simulink model "Lab2_TopolnitskiiA_R31342020c_slx"  (R2020b)
settings: Solver=VariableStepAuto  StartTime=0.0  StopTime=10.0  RelTol=1e-3
libraries: roblocks x4, simulink x3
settings Model: Creator=Insight  LastModifiedBy=Insight
settings DebuggingCC: SFMachineParentedDataDiag=error

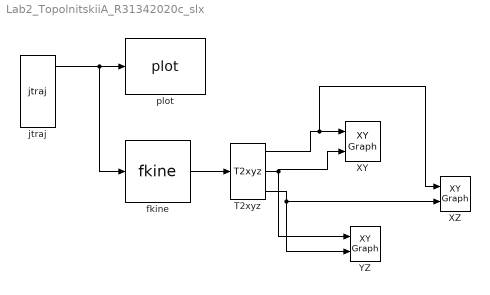
== system Lab2_TopolnitskiiA_R31342020c_slx ==
  T2xyz : roblocks/Toolbox/T2xyz
  XY : simulink/Sinks/XY Graph  xmin=-1  xmax=1  ymin=-1  ymax=1  st=-1
  XZ : simulink/Sinks/XY Graph  xmin=-1.5  xmax=1.5  ymin=-1.5  ymax=1.5  st=-1
  "YZ " : simulink/Sinks/XY Graph  xmin=-1.5  xmax=1.5  ymin=-1.5  ymax=1.5  st=-1
  fkine : roblocks/Arm/fkine  robot=irb140
  jtraj : roblocks/Toolbox/jtraj  q0=[pi/4 pi/4 pi/10 pi/10 pi/15 pi/5]  qf=[-pi/4 -6*pi/7 pi/2 -pi -pi/3 -2*pi/3]  tmax=3  ts=0.02
  plot : roblocks/Arm/plot  robot=irb140  fps=5  holdplot=on
  wires:
  jtraj/1 -> fkine/1, plot/1
  fkine/1 -> T2xyz/1
  T2xyz/1 -> XZ/1, XY/1
  T2xyz/2 -> "YZ "/1, XY/2
  T2xyz/3 -> XZ/2, "YZ "/2
